simulink library "BLE_Library"  (R2017b)
settings: Solver=VariableStepAuto  StartTime=0.0  StopTime=10.0  RelTol=1e-3
values from neighbouring files (symbols this model uses):
  D = D/ScaleCoefficient    [BLE_PostLoad.m]    (also in new_BLE_model.m = zeros(N_BLE,N_BLE+1))
undefined symbols (not defined in the file or in its folder): ADV_IND_AccA, ADV_IND_id, BT_Hop_Separation, BT_Samples_Per_Symbol, CONNECT_IND_id, CONNECT_IND_length, F3B672D172DF, F506B10B1B3E, Header, LL_DATA_EMPTY_length, LL_DATA_id, magnitude, Payload, Preamble, Slot_Ts, T_IFS
libraries: BLE_Library x56, simulink x39, commutil2 x29, dspindex x17, commdigbbndfm2 x5, dspsigops x2, commrandsrc3 x2, dspstat3 x2, dspsrcs4 x1, dsparch4 x1, commdigbbndcpm2 x1
(part 2 of 5)

== system BLE_Library/CRC, Whitening, Modulation ==
  "Preamble, Access" : Inport
  "Header, Payload" : Inport  Port=2
  CRC_ini : Inport  Port=3
  ChIdx : Inport  Port=4
  Enable : EnablePort  StatesWhenEnabling=reset  ShowOutputPort=on
  CRC calculation : Subsystem  TreatAsAtomicUnit=on
  Compare To Constant : simulink/Logic and Bit Operations/Compare To Constant  relop=>  const=39  OutDataTypeStr=boolean
  Concatenate : Concatenate  Mode=Multidimensional array
  Counter Free-Running : simulink/Sources/Counter Free-Running  NumBits=32  tsamp=Slot_Ts
  Logical Operator1 : Logic  AllPortsSameDT=off  OutDataTypeStr=boolean
  Logical Operator2 : Logic  Operator=NOT  AllPortsSameDT=off  OutDataTypeStr=boolean
  Modulation : Subsystem
  Relational Operator1 : RelationalOperator  Operator=>  OutDataTypeStr=boolean  RndMeth=Simplest
  Selector1 : Subsystem
  Selector2 : Subsystem  TreatAsAtomicUnit=on
  Switch : Switch  Criteria=u2 > Threshold
  Switch1 : Switch  Criteria=u2 > Threshold
  Vector Concatenate1 : Concatenate
  Whitening : Subsystem
  Width1 : Width
  add CRC length : Bias  Bias=24
  TxBits : Outport  OutputWhenDisabled=reset  InitialOutput=0
  TxBitsLength : Outport  Port=2
  Tx signal : Outport  Port=3  OutputWhenDisabled=reset  InitialOutput=0
  wires:
  CRC_ini/1 -> CRC calculation/2(CRC_ini)
  "Preamble, Access"/1 -> Concatenate/1
  ChIdx/1 -> Whitening/2(ChIdx), Modulation/2(ChIdx)
  Counter Free-Running/1 -> Relational Operator1/2, Compare To Constant/1, Selector1/2(Idx)
  Concatenate/1 -> Width1/1, Selector1/1(U)
  "Header, Payload"/1 -> Concatenate/2
  Compare To Constant/1 -> Switch1/2, Whitening/Enable, Logical Operator1/2
  Width1/1 -> add CRC length/1, Relational Operator1/1
  Relational Operator1/1 -> Switch/2, Logical Operator2/1, Logical Operator1/1, Selector1/Enable
  Modulation/1(TxBits) -> Vector Concatenate1/1
  CRC calculation/1(CRC) -> Selector2/1(U)
  Switch1/1 -> Modulation/1(Tx bits)
  Enable/1 -> Vector Concatenate1/2
  Selector1/1(Out1) -> Switch1/3, Switch/1, CRC calculation/1(Payload)
  Logical Operator1/1 -> CRC calculation/Enable
  Selector2/1(Out1) -> Switch/3
  Logical Operator2/1 -> Selector2/Enable
  Modulation/2(Tx signal) -> Tx signal/1
  Vector Concatenate1/1 -> TxBits/1
  add CRC length/1 -> TxBitsLength/1
  Switch/1 -> Whitening/1(Payload)
  Whitening/1(Payload W) -> Switch1/1

== system BLE_Library/Channel ==

== system BLE_Library/Demodulation, De-whitening, CRC check, PDU ==
  Rx signal : Inport
  CRC_ini : Inport  Port=2
  AccA : Inport  Port=3
  ChIdx : Inport  Port=4
  Enable : EnablePort  StatesWhenEnabling=reset
  "Access Code check, Payload read enable" : Subsystem
  "De-whitening, CRC check, Data fields" : Subsystem
  Demodulation : Subsystem
  Terminator : Terminator
  AccA_OK : Outport
  CRC_OK : Outport  Port=2
  Payload_En : Outport  Port=3
  Header : Outport  Port=4
  PDU : Outport  Port=5
  RxBits : Outport  Port=6
  wires:
  "De-whitening, CRC check, Data fields"/3(PDU) -> PDU/1
  ChIdx/1 -> Demodulation/2(ChIdx), "De-whitening, CRC check, Data fields"/3(ChIdx)
  Demodulation/3(Rx bit 0) -> Terminator/1
  "De-whitening, CRC check, Data fields"/1(CRC_OK) -> CRC_OK/1
  Demodulation/1(Rx bit detected) -> "Access Code check, Payload read enable"/1(Rx bit detected)
  Demodulation/2(Rx bit 1) -> RxBits/1, "Access Code check, Payload read enable"/2(Rx bit 1), "De-whitening, CRC check, Data fields"/1(Paylaod W)
  Rx signal/1 -> Demodulation/1(Rx signal)
  "Access Code check, Payload read enable"/1(PayloadEn) -> "De-whitening, CRC check, Data fields"/Enable, Payload_En/1
  CRC_ini/1 -> "De-whitening, CRC check, Data fields"/2(CRC_ini)
  AccA/1 -> "Access Code check, Payload read enable"/3(AccA)
  "Access Code check, Payload read enable"/2(AccA_OK) -> AccA_OK/1
  "De-whitening, CRC check, Data fields"/2(Header) -> Header/1

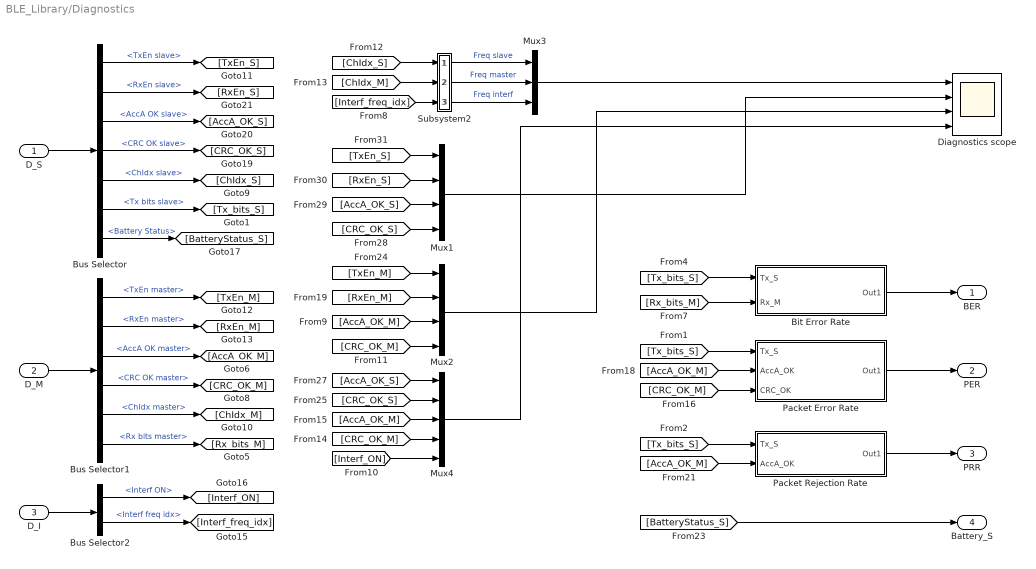
== system BLE_Library/Diagnostics ==
  D_S : Inport
  D_M : Inport  Port=2
  D_I : Inport  Port=3
  Bit Error Rate : Subsystem
      mask Display: disp('BER\n calculation')
  Bus Selector : BusSelector  OutputSignals=TxEn slave,RxEn slave,AccA OK slave,CRC OK slave,ChIdx slave,Tx bits slave,Battery Status
  Bus Selector1 : BusSelector  OutputSignals=TxEn master,RxEn master,AccA OK master,CRC OK master,ChIdx master,Rx bits master
  Bus Selector2 : BusSelector  OutputSignals=Interf ON,Interf freq idx
  Diagnostics scope : Scope  NumInputPorts=4
  Mux1 : Mux
  Mux2 : Mux
  Mux3 : Mux  Inputs=3
  Mux4 : Mux  Inputs=5
  Packet Error Rate : Subsystem
      mask Display: disp('PER\n calculation')
  Packet Rejection Rate : Subsystem
      mask Display: disp('PRR\n calculation')
  Subsystem2 : Subsystem
      mask Display: disp('')
  BER : Outport
  PER : Outport  Port=2
  PRR : Outport  Port=3
  Battery_S : Outport  Port=4
  wires:
  Mux4/1 -> Diagnostics scope/4
  Mux2/1 -> Diagnostics scope/3
  Mux1/1 -> Diagnostics scope/2
  Mux3/1 -> Diagnostics scope/1
  D_S/1 -> Bus Selector/1
  D_M/1 -> Bus Selector1/1
  Bit Error Rate/1(Out1) -> BER/1
  Bus Selector/6 -> [Tx_bits_S]  "<Tx bits slave>"
  [Tx_bits_S] -> Bit Error Rate/1(Tx_S)
  Bus Selector1/6 -> [Rx_bits_M]  "<Rx bits master>"
  [Rx_bits_M] -> Bit Error Rate/2(Rx_M)
  Bus Selector1/3 -> [AccA_OK_M]  "<AccA OK master>"
  Bus Selector1/4 -> [CRC_OK_M]  "<CRC OK master>"
  Bus Selector/5 -> [ChIdx_S]  "<ChIdx slave>"
  Bus Selector1/5 -> [ChIdx_M]  "<ChIdx master>"
  [CRC_OK_M] -> Mux4/4
  [AccA_OK_M] -> Packet Error Rate/2(AccA_OK)
  [CRC_OK_M] -> Packet Error Rate/3(CRC_OK)
  Packet Rejection Rate/1(Out1) -> PRR/1
  Bus Selector1/2 -> [RxEn_M]  "<RxEn master>"
  [RxEn_M] -> Mux2/2
  [AccA_OK_M] -> Packet Rejection Rate/2(AccA_OK)
  Packet Error Rate/1(Out1) -> PER/1
  [AccA_OK_M] -> Mux4/3
  [Interf_ON] -> Mux4/5
  [AccA_OK_M] -> Mux2/3
  [CRC_OK_M] -> Mux2/4
  [ChIdx_S] -> Subsystem2/1(In1)
  [ChIdx_M] -> Subsystem2/2(In2)
  [Interf_freq_idx] -> Subsystem2/3(In3)
  Subsystem2/1(Out1) -> Mux3/1  "Freq slave"
  Subsystem2/2(Out2) -> Mux3/2  "Freq master"
  Subsystem2/3(Out3) -> Mux3/3  "Freq interf"
  D_I/1 -> Bus Selector2/1
  Bus Selector2/1 -> [Interf_ON]  "<Interf ON>"
  Bus Selector2/2 -> [Interf_freq_idx]  "<Interf freq idx>"
  Bus Selector1/1 -> [TxEn_M]  "<TxEn master>"
  [TxEn_M] -> Mux2/1
  Bus Selector/4 -> [CRC_OK_S]  "<CRC OK slave>"
  [CRC_OK_S] -> Mux4/2
  Bus Selector/3 -> [AccA_OK_S]  "<AccA OK slave>"
  [AccA_OK_S] -> Mux4/1
  Bus Selector/2 -> [RxEn_S]  "<RxEn slave>"
  Bus Selector/1 -> [TxEn_S]  "<TxEn slave>"
  [AccA_OK_S] -> Mux1/3
  [CRC_OK_S] -> Mux1/4
  [RxEn_S] -> Mux1/2
  [TxEn_S] -> Mux1/1
  Bus Selector/7 -> [BatteryStatus_S]  "<Battery Status>"
  [BatteryStatus_S] -> Battery_S/1
  [Tx_bits_S] -> Packet Error Rate/1(Tx_S)
  [Tx_bits_S] -> Packet Rejection Rate/1(Tx_S)

== system BLE_Library/Export parameters ==

== system BLE_Library/Falling edge ==
  In1 : Inport
  Logical Operator3 : Logic  Operator=XOR  AllPortsSameDT=off  OutDataTypeStr=boolean
  Logical Operator4 : Logic  AllPortsSameDT=off  OutDataTypeStr=boolean
  Unit Delay1 : UnitDelay  SampleTime=Slot_Ts
  Out1 : Outport
  wires:
  In1/1 -> Logical Operator3/1, Unit Delay1/1
  Logical Operator4/1 -> Out1/1
  Unit Delay1/1 -> Logical Operator4/2, Logical Operator3/2
  Logical Operator3/1 -> Logical Operator4/1

== system BLE_Library/Packet Error Rate ==
  Tx_S : Inport
  AccA_OK : Inport  Port=2
  CRC_OK : Inport  Port=3
  Compare To Zero : simulink/Logic and Bit Operations/Compare To Zero  relop=>  OutDataTypeStr=boolean
  Constant : Constant  SampleTime=Slot_Ts
  Demux1 : Demux  Outputs=2
  Divide : Product  Inputs=*/
  Enabled Subsystem : Subsystem  TreatAsAtomicUnit=on
  Falling edge : BLE_Library/Falling edge  SystemSampleTime=-1
  Logical Operator : Logic  AllPortsSameDT=off  OutDataTypeStr=boolean
  Logical Operator2 : Logic  AllPortsSameDT=off  OutDataTypeStr=boolean
  Logical Operator3 : Logic  AllPortsSameDT=off  OutDataTypeStr=boolean
  Subsystem1 : BLE_Library/Subsystem2  offset=0
  Subsystem4 : BLE_Library/Subsystem2  offset=0
  Sum : Sum  Inputs=|-+
  Switch : Switch  Criteria=u2 > Threshold
  Terminator1 : Terminator
  Unit Delay1 : UnitDelay  SampleTime=Slot_Ts
  Unit Delay2 : UnitDelay  SampleTime=Slot_Ts
  Vector Concatenate1 : Concatenate  NumInputs=3
  Out1 : Outport
  wires:
  Constant/1 -> Switch/3
  Switch/1 -> Divide/2
  Compare To Zero/1 -> Logical Operator/2
  Logical Operator/1 -> Enabled Subsystem/Enable
  Falling edge/1 -> Logical Operator/1
  Sum/1 -> Divide/1, Vector Concatenate1/2
  Subsystem4/1 -> Sum/1
  Divide/1 -> Vector Concatenate1/1
  Subsystem1/1 -> Sum/2, Vector Concatenate1/3, Switch/1, Compare To Zero/1, Switch/2
  Vector Concatenate1/1 -> Enabled Subsystem/1(In1)
  Enabled Subsystem/1(Out1) -> Out1/1
  Tx_S/1 -> Unit Delay1/1
  Logical Operator2/1 -> Subsystem1/1
  Logical Operator3/1 -> Subsystem4/1
  Unit Delay2/1 -> Logical Operator2/2, Logical Operator3/1
  CRC_OK/1 -> Logical Operator3/2
  AccA_OK/1 -> Logical Operator2/1
  Unit Delay1/1 -> Demux1/1
  Demux1/1 -> Terminator1/1
  Demux1/2 -> Falling edge/1, Unit Delay2/1

== system BLE_Library/Packet Rejection Rate ==
  Tx_S : Inport
  AccA_OK : Inport  Port=2
  Compare To Zero1 : simulink/Logic and Bit Operations/Compare To Zero  relop=>  OutDataTypeStr=boolean
  Constant : Constant  SampleTime=Slot_Ts
  Demux : Demux  Outputs=2
  Divide1 : Product  Inputs=*/
  Enabled Subsystem1 : Subsystem  TreatAsAtomicUnit=on
  Falling edge : BLE_Library/Falling edge  SystemSampleTime=-1
  Logical Operator1 : Logic  AllPortsSameDT=off  OutDataTypeStr=boolean
  Logical Operator3 : Logic  AllPortsSameDT=off  OutDataTypeStr=boolean
  Rising edge : BLE_Library/Rising edge  SystemSampleTime=-1
  Subsystem1 : BLE_Library/Subsystem2  offset=0
  Subsystem4 : BLE_Library/Subsystem2  offset=0
  Sum1 : Sum  Inputs=|-+
  Switch : Switch  Criteria=u2 > Threshold
  Terminator : Terminator
  Unit Delay1 : UnitDelay  SampleTime=Slot_Ts
  Unit Delay2 : UnitDelay  SampleTime=Slot_Ts
  Vector Concatenate2 : Concatenate  NumInputs=3
  Out1 : Outport
  wires:
  Demux/2 -> Unit Delay1/1
  Demux/1 -> Terminator/1
  Tx_S/1 -> Demux/1
  Rising edge/1 -> Subsystem1/1
  Logical Operator3/1 -> Subsystem4/1
  AccA_OK/1 -> Logical Operator3/2
  Unit Delay2/1 -> Logical Operator3/1
  Unit Delay1/1 -> Rising edge/1, Unit Delay2/1, Falling edge/1
  Switch/1 -> Divide1/2
  Constant/1 -> Switch/3
  Compare To Zero1/1 -> Logical Operator1/2
  Vector Concatenate2/1 -> Enabled Subsystem1/1(In1)
  Divide1/1 -> Vector Concatenate2/1
  Subsystem1/1 -> Switch/2, Compare To Zero1/1, Switch/1, Vector Concatenate2/3, Sum1/2
  Falling edge/1 -> Logical Operator1/1
  Subsystem4/1 -> Sum1/1
  Sum1/1 -> Vector Concatenate2/2, Divide1/1
  Logical Operator1/1 -> Enabled Subsystem1/Enable
  Enabled Subsystem1/1(Out1) -> Out1/1

== system BLE_Library/Rising edge ==
  In1 : Inport
  Logical Operator3 : Logic  Operator=XOR  AllPortsSameDT=off  OutDataTypeStr=boolean
  Logical Operator4 : Logic  AllPortsSameDT=off  OutDataTypeStr=boolean
  Unit Delay1 : UnitDelay  SampleTime=Slot_Ts
  Out1 : Outport
  wires:
  In1/1 -> Logical Operator4/1, Logical Operator3/1, Unit Delay1/1
  Logical Operator4/1 -> Out1/1
  Unit Delay1/1 -> Logical Operator3/2
  Logical Operator3/1 -> Logical Operator4/2

== system BLE_Library/Sensor ==
  Integer to Bit Converter : commutil2/Integer to Bit Converter  nbits=NbitsPerSample  signedInputValues=Unsigned  bitOrder=MSB first  outDtype=boolean
  Rounding Function : Rounding  Operator=round
  Uniform Random Number : UniformRandomNumber  Minimum=0  Maximum=2^NbitsPerSample-1  SampleTime=Slot_Ts
  Out1 : Outport
  wires:
  Uniform Random Number/1 -> Rounding Function/1
  Rounding Function/1 -> Integer to Bit Converter/1
  Integer to Bit Converter/1 -> Out1/1

== system BLE_Library/Subsystem1 ==
  En_in : Inport
  PDU_type : Inport  Port=2
  Constant5 : Constant  Value=PDU_type  SampleTime=Slot_Ts
  Logical Operator3 : Logic  AllPortsSameDT=off  OutDataTypeStr=boolean
  Relational Operator3 : RelationalOperator  Operator===  OutDataTypeStr=boolean  RndMeth=Simplest
  En_out : Outport
  wires:
  PDU_type/1 -> Relational Operator3/2
  Logical Operator3/1 -> En_out/1
  Constant5/1 -> Relational Operator3/1
  En_in/1 -> Logical Operator3/1
  Relational Operator3/1 -> Logical Operator3/2

== system BLE_Library/Subsystem2 ==
  <CRC OK slave> : Inport
  Add1 : Sum  AccumDataTypeStr=uint32
  Add2 : Sum  Inputs=+-
  Constant : Constant  Value=offset  SampleTime=Slot_Ts
  Data Type Conversion1 : DataTypeConversion  OutDataTypeStr=double
  Unit Delay1 : UnitDelay  SampleTime=Slot_Ts
  Out1 : Outport
  wires:
  <CRC OK slave>/1 -> Data Type Conversion1/1
  Unit Delay1/1 -> Add1/1
  Add1/1 -> Add2/1, Unit Delay1/1
  Data Type Conversion1/1 -> Add1/2
  Add2/1 -> Out1/1
  Constant/1 -> Add2/2

== system BLE_Library/802.11b interferer/Enabled Subsystem ==
  In1 : Inport
  Enable : EnablePort  StatesWhenEnabling=reset
  Out3 : Outport  OutputWhenDisabled=reset  InitialOutput=0
  wires:
  In1/1 -> Out3/1

== system BLE_Library/802.11b interferer/Poisson pulses ==
  Constant5 : Constant  Value=1/average_rate-packet_length  SampleTime=Slot_Ts
  Constant6 : Constant  Value=0  SampleTime=Slot_Ts
  If : If  IfExpression=u1
  If Action Subsystem1 : Subsystem  TreatAsAtomicUnit=on
  If Action Subsystem2 : Subsystem  TreatAsAtomicUnit=on
  Merge : Merge
  Relational Operator1 : RelationalOperator  Operator=<=  OutDataTypeStr=boolean  RndMeth=Simplest
  enable : Outport
  wires:
  Constant6/1 -> Relational Operator1/2
  If/2 -> If Action Subsystem1/Action
  If/1 -> If Action Subsystem2/Action
  Relational Operator1/1 -> If/1
  Constant5/1 -> Relational Operator1/1
  If Action Subsystem2/1(enable) -> Merge/1
  If Action Subsystem1/1(enable) -> Merge/2
  Merge/1 -> enable/1

== system BLE_Library/BLE master/Master mode ==
  note: 1) Add Subsystem or Model blocks as valid variant choices.
      | 2) You cannot connect blocks at this level. At simulation, connectivity is automatically
      | determined, based on the active variant and port name matching.
  Turn ON : Inport
  Rx signal : Inport  Port=2
  In3 : Inport  Port=3
  Multiple slaves mode : Subsystem  VariantControl=MultipleSlavesMode
  One slave mode : Subsystem  VariantControl=OneSlaveMode
  Tx signal : Outport
  Diagnostics : Outport  Port=2

== system BLE_Library/BLE master/Subsystem7 ==
  In1 : Inport
  Compare To Zero : simulink/Logic and Bit Operations/Compare To Zero  relop=>  OutDataTypeStr=boolean
  Constant4 : Constant  Value=zeros(BT_Samples_Per_Symbol,1)  SampleTime=Slot_Ts
  Real-Imag to Complex : RealImagToComplex
  Step : Step  Time=3.492e-3  Before=1  After=0  SampleTime=Slot_Ts
  Step1 : Step  Time=3.55e-3  SampleTime=Slot_Ts
  Step2 : Step  Time=4060e-3  SampleTime=Slot_Ts
  Step5 : Step  Time=4020e-3  SampleTime=Slot_Ts
  Sum1 : Sum  Inputs=++-+
  Switch : Switch  Criteria=u2 > Threshold
  Out1 : Outport
  Out2 : Outport  Port=2
  wires:
  Compare To Zero/1 -> Out2/1
  Sum1/1 -> Switch/2, Compare To Zero/1
  Step/1 -> Sum1/1
  Step5/1 -> Sum1/3
  Step1/1 -> Sum1/2
  Switch/1 -> Out1/1
  In1/1 -> Switch/1
  Real-Imag to Complex/1 -> Switch/3
  Constant4/1 -> Real-Imag to Complex/2, Real-Imag to Complex/1
  Step2/1 -> Sum1/4

== system BLE_Library/BLE slave/ADV_IND ==
  Enable : EnablePort  StatesWhenEnabling=reset
  "ADV_IND Header, Payload" : Subsystem
  Subsystem4 : Subsystem
      mask Display: disp('Adv\nPreamble,\nAccess')
  "Preamble, Access" : Outport  InitialOutput=0
  "Header, Payload" : Outport  Port=2  InitialOutput=0
  wires:
  "ADV_IND Header, Payload"/1("Header, Payload") -> "Header, Payload"/1
  Subsystem4/1(Out1) -> "Preamble, Access"/1

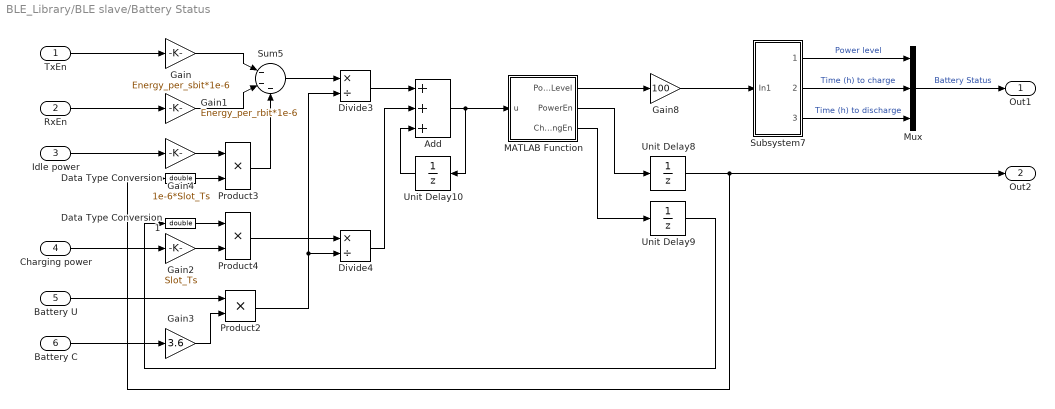
== system BLE_Library/BLE slave/Battery Status ==
  TxEn : Inport
  RxEn : Inport  Port=2
  Idle power : Inport  Port=3
  Charging power : Inport  Port=4
  Battery U : Inport  Port=5
  Battery C : Inport  Port=6
  Add : Sum  Inputs=+++
  Data Type Conversion : DataTypeConversion  OutDataTypeStr=double
  Data Type Conversion1 : DataTypeConversion  OutDataTypeStr=double
  Divide3 : Product  Inputs=*/
  Divide4 : Product  Inputs=*/
  Gain : Gain  Gain=Energy_per_sbit*1e-6
  Gain1 : Gain  Gain=Energy_per_rbit*1e-6
  Gain2 : Gain  Gain=Slot_Ts
  Gain3 : Gain  Gain=3.6
  Gain4 : Gain  Gain=1e-6*Slot_Ts
  Gain8 : Gain  Gain=100
  MATLAB Function : MATLAB Function  TreatAsAtomicUnit=on
  Mux : Mux  Inputs=3
  Product2 : Product
  Product3 : Product
  Product4 : Product
  Subsystem7 : Subsystem
      mask Display: disp('Battery\nStatus')
  Sum5 : Sum  Inputs=|---
  Unit Delay10 : UnitDelay  InitialCondition=1  SampleTime=Slot_Ts
  Unit Delay8 : UnitDelay  SampleTime=Slot_Ts
  Unit Delay9 : UnitDelay  SampleTime=Slot_Ts
  Out1 : Outport
  Out2 : Outport  Port=2
  wires:
  Mux/1 -> Out1/1  "Battery Status"
  TxEn/1 -> Gain/1
  RxEn/1 -> Gain1/1
  Idle power/1 -> Gain4/1
  Product3/1 -> Sum5/3
  Product2/1 -> Divide4/2, Divide3/2
  Battery U/1 -> Product2/1
  Gain4/1 -> Product3/1
  Battery C/1 -> Gain3/1
  Gain3/1 -> Product2/2
  Unit Delay8/1 -> Out2/1, Data Type Conversion/1
  Data Type Conversion/1 -> Product3/2
  Gain8/1 -> Subsystem7/1(In1)
  MATLAB Function/2(PowerEn) -> Unit Delay8/1
  MATLAB Function/3(ChargingEn) -> Unit Delay9/1
  Charging power/1 -> Gain2/1
  Gain/1 -> Sum5/1
  Gain1/1 -> Sum5/2
  Unit Delay9/1 -> Data Type Conversion1/1
  Sum5/1 -> Divide3/1
  Product4/1 -> Divide4/1
  MATLAB Function/1(PowerLevel) -> Gain8/1
  Data Type Conversion1/1 -> Product4/1
  Gain2/1 -> Product4/2
  Divide3/1 -> Add/1
  Divide4/1 -> Add/2
  Add/1 -> Unit Delay10/1, MATLAB Function/1(u)
  Unit Delay10/1 -> Add/3
  Subsystem7/3(Time (h) to discharge) -> Mux/3  "Time (h) to discharge"
  Subsystem7/2(Time (h) to charge) -> Mux/2  "Time (h) to charge"
  Subsystem7/1(Power level) -> Mux/1  "Power level"

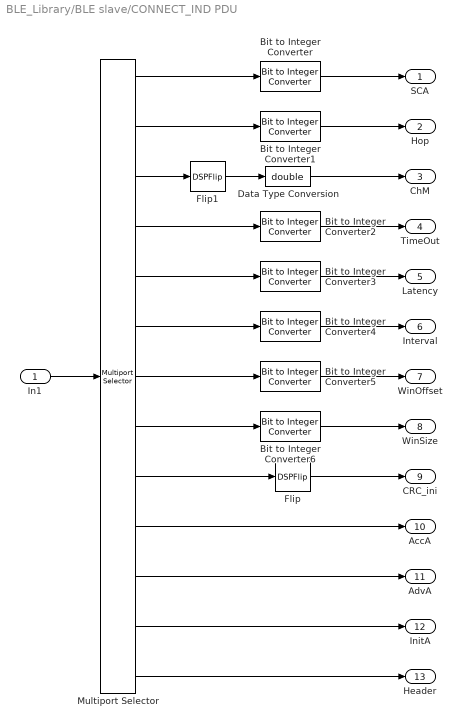
== system BLE_Library/BLE slave/CONNECT_IND PDU ==
  In1 : Inport  OutDataTypeStr=boolean
  Bit to Integer Converter : commutil2/Bit to Integer Converter  nbits=3  bitOrder=MSB first  signedOutputValues=Unsigned  outDtype=double  outDtypeSigned=Inherit via internal rule
  Bit to Integer Converter1 : commutil2/Bit to Integer Converter  nbits=5  bitOrder=MSB first  signedOutputValues=Unsigned  outDtype=double  outDtypeSigned=Inherit via internal rule
  Bit to Integer Converter{2..5} (4 alike) : commutil2/Bit to Integer Converter  nbits=16  bitOrder=MSB first  signedOutputValues=Unsigned  outDtype=double  outDtypeSigned=Inherit via internal rule
  Bit to Integer Converter6 : commutil2/Bit to Integer Converter  nbits=8  bitOrder=MSB first  signedOutputValues=Unsigned  outDtype=double  outDtypeSigned=Inherit via internal rule
  Data Type Conversion : DataTypeConversion  OutDataTypeStr=double
  Flip : DSPFlip
  Flip1 : DSPFlip
  Multiport Selector : dspindex/Multiport Selector  rowsOrCols=Rows  idxCellArray={1:3,4:8,9:48,49:64,65:80,81:96,97:112,113:120,121:144,145:176,177:224,225:272,273:288}  idxErrMode=Clip Index
  SCA : Outport
  Hop : Outport  Port=2
  ChM : Outport  Port=3
  TimeOut : Outport  Port=4
  Latency : Outport  Port=5
  Interval : Outport  Port=6
  WinOffset : Outport  Port=7
  WinSize : Outport  Port=8
  CRC_ini : Outport  Port=9
  AccA : Outport  Port=10
  AdvA : Outport  Port=11
  InitA : Outport  Port=12
  Header : Outport  Port=13
  wires:
  Flip1/1 -> Data Type Conversion/1
  Flip/1 -> CRC_ini/1
  Data Type Conversion/1 -> ChM/1
  Bit to Integer Converter6/1 -> WinSize/1
  Bit to Integer Converter5/1 -> WinOffset/1
  Bit to Integer Converter4/1 -> Interval/1
  Bit to Integer Converter3/1 -> Latency/1
  Bit to Integer Converter2/1 -> TimeOut/1
  Bit to Integer Converter1/1 -> Hop/1
  Bit to Integer Converter/1 -> SCA/1
  Multiport Selector/13 -> Header/1
  Multiport Selector/12 -> InitA/1
  Multiport Selector/11 -> AdvA/1
  Multiport Selector/10 -> AccA/1
  Multiport Selector/9 -> Flip/1
  Multiport Selector/8 -> Bit to Integer Converter6/1
  Multiport Selector/7 -> Bit to Integer Converter5/1
  Multiport Selector/6 -> Bit to Integer Converter4/1
  Multiport Selector/5 -> Bit to Integer Converter3/1
  Multiport Selector/4 -> Bit to Integer Converter2/1
  Multiport Selector/3 -> Flip1/1
  Multiport Selector/2 -> Bit to Integer Converter1/1
  Multiport Selector/1 -> Bit to Integer Converter/1
  In1/1 -> Multiport Selector/1

== system BLE_Library/BLE slave/LL_DATA ==
  Access : Inport
  MD_SN_NESN : Inport  Port=2
  Data : Inport  Port=3
  Enable : EnablePort  StatesWhenEnabling=reset
  "Concatenate Preamble, Access address" : Concatenate  Mode=Multidimensional array
  Fcn : Fcn  Expr=u/8
  Flip : DSPFlip
  Flip1 : DSPFlip
  Header : Concatenate  NumInputs=4  Mode=Multidimensional array
  Header and Payload : Concatenate  Mode=Multidimensional array
  Integer to Bit Converter3 : commutil2/Integer to Bit Converter  nbits=8  signedInputValues=Unsigned  bitOrder=MSB first  outDtype=boolean
  LLID : Constant  Value=[0 1]'  OutDataTypeStr=boolean  SampleTime=Slot_Ts
  MATLAB Function : MATLAB Function  TreatAsAtomicUnit=on
  RFU : Constant  Value=[0 0 0]'  OutDataTypeStr=boolean  SampleTime=Slot_Ts
  Width : Width
  "Preamble, Access" : Outport  InitialOutput=0
  "Header, Payload" : Outport  Port=2  InitialOutput=0
  wires:
  Data/1 -> Header and Payload/2, Width/1
  Flip1/1 -> Header/4
  RFU/1 -> Header/3
  Flip/1 -> Header/2
  MD_SN_NESN/1 -> Flip/1
  Header/1 -> Header and Payload/1
  Header and Payload/1 -> "Header, Payload"/1
  Integer to Bit Converter3/1 -> Flip1/1
  Width/1 -> Fcn/1
  Fcn/1 -> Integer to Bit Converter3/1
  LLID/1 -> Header/1
  "Concatenate Preamble, Access address"/1 -> "Preamble, Access"/1
  MATLAB Function/1(Preamble) -> "Concatenate Preamble, Access address"/1
  Access/1 -> MATLAB Function/1(AccessAddress), "Concatenate Preamble, Access address"/2

== system BLE_Library/BLE slave/Subsystem ==
  Data in : Inport
  Enable : EnablePort  StatesWhenEnabling=reset
  Data out : Outport
  wires:
  Data in/1 -> Data out/1

== system BLE_Library/BLE slave/Subsystem3 ==
  In1 : Inport
  Constant4 : Constant  Value=zeros(BT_Samples_Per_Symbol,1)  SampleTime=Slot_Ts
  Real-Imag to Complex : RealImagToComplex
  Step2 : Step  Time=10e-3  Before=1  After=0  SampleTime=Slot_Ts
  Step3 : Step  Time=3500  SampleTime=Slot_Ts
  Sum2 : Sum  Inputs=|++
  Switch : Switch  Criteria=u2 > Threshold
  Out1 : Outport
  wires:
  Constant4/1 -> Real-Imag to Complex/1, Real-Imag to Complex/2
  Real-Imag to Complex/1 -> Switch/3
  Step3/1 -> Sum2/1
  Step2/1 -> Sum2/2
  Sum2/1 -> Switch/2
  In1/1 -> Switch/1
  Switch/1 -> Out1/1

== system BLE_Library/BLE slave/Subsystem5 ==
  AdvA : Inport
  InitA : Inport  Port=2
  Compare To Constant1 : simulink/Logic and Bit Operations/Compare To Constant  relop===  const=1  OutDataTypeStr=boolean
  Constant1 : Constant  Value=PDU_Type  VectorParams1D=off  OutDataTypeStr=double  SampleTime=Slot_Ts
  If : If  IfExpression=u1
  If Action Subsystem : Subsystem  TreatAsAtomicUnit=on
  If Action Subsystem1 : Subsystem  TreatAsAtomicUnit=on
  Merge2 : Merge
  CON OK : Outport
  wires:
  If/2 -> If Action Subsystem1/Action
  AdvA/1 -> If Action Subsystem1/1(AdvA), If Action Subsystem/1(AdvA)
  InitA/1 -> If Action Subsystem1/2(InitA)
  If/1 -> If Action Subsystem/Action
  If Action Subsystem1/1(CON OK) -> Merge2/2
  If Action Subsystem/1(CON OK) -> Merge2/1
  Merge2/1 -> CON OK/1
  Constant1/1 -> Compare To Constant1/1
  Compare To Constant1/1 -> If/1

== system BLE_Library/BLE slave/Subsystem7 ==
  In1 : Inport
  Compare To Zero : simulink/Logic and Bit Operations/Compare To Zero  relop=>  OutDataTypeStr=boolean
  Constant4 : Constant  Value=zeros(BT_Samples_Per_Symbol,1)  SampleTime=Slot_Ts
  Real-Imag to Complex : RealImagToComplex
  Step : Step  Time=3.74e-3  Before=1  After=0  SampleTime=Slot_Ts
  Step1 : Step  Time=3.75e-3  SampleTime=Slot_Ts
  Step2 : Step  Time=4.78e-3  SampleTime=Slot_Ts
  Step5 : Step  Time=4.16e-3  SampleTime=Slot_Ts
  Sum1 : Sum  Inputs=++-+
  Switch : Switch  Criteria=u2 > Threshold
  Out1 : Outport
  Out2 : Outport  Port=2
  wires:
  Constant4/1 -> Real-Imag to Complex/1, Real-Imag to Complex/2
  Real-Imag to Complex/1 -> Switch/3
  In1/1 -> Switch/1
  Switch/1 -> Out1/1
  Step1/1 -> Sum1/2
  Step5/1 -> Sum1/3
  Step/1 -> Sum1/1
  Sum1/1 -> Compare To Zero/1, Switch/2
  Compare To Zero/1 -> Out2/1
  Step2/1 -> Sum1/4

== system BLE_Library/Bit Error Rate/Enabled Subsystem1 ==
  In1 : Inport
  Enable : EnablePort
  Out1 : Outport
  wires:
  In1/1 -> Out1/1

== system BLE_Library/CRC, Whitening, Modulation/CRC calculation ==
  Payload : Inport
  CRC_ini : Inport  Port=2
  Enable : EnablePort  StatesWhenEnabling=reset
  CRC generation : MATLAB Function  TreatAsAtomicUnit=on
  Constant3 : Constant  SampleTime=Slot_Ts
  Flip : DSPFlip
  Switch : Switch  Criteria=u2 > Threshold
  Unit Delay1 : UnitDelay  SampleTime=Slot_Ts
  Unit Delay8 : UnitDelay  SampleTime=Slot_Ts
  CRC : Outport
  wires:
  Payload/1 -> CRC generation/1(bin)
  Unit Delay1/1 -> Switch/2
  Constant3/1 -> Unit Delay1/1
  CRC generation/1(CRC) -> Unit Delay8/1, Flip/1
  CRC_ini/1 -> Switch/3
  Unit Delay8/1 -> Switch/1
  Switch/1 -> CRC generation/2(LFSR)
  Flip/1 -> CRC/1

== system BLE_Library/CRC, Whitening, Modulation/Modulation ==
  Tx bits : Inport
  ChIdx : Inport  Port=2
  GFSK Modulation : commdigbbndcpm2/CPM Modulator Baseband  Mnum=2  inputType=Bit  mappingType=Binary  modIdx=0.5  pulseShape=Gaussian  BT=0.5  mainLobePulseLength=1  rollOff=0.2  pulseLength=1  preHistory=1  phaseOffset=0  samplesPerSymbol=BT_Samples_Per_Symbol  RateOptions=Enforce single-rate processing  outDataType=double
      settings: SourceProductName=Communications System Toolbox  SourceProductBaseCode=CM
  Look-Up Table : Lookup  InputValues=0:39  Table=[1:11 13:38 0 12 39]  SaturateOnIntegerOverflow=on
  M-FSK Modulator Baseband : commdigbbndfm2/M-FSK Modulator Baseband  M=Num_Hop_Frequencies  InType=Integer  Enc=Binary  freqSep=BT_Hop_Separation  phaseType=Continuous  numSamp=BT_Samples_Per_Symbol  RateOptions=Enforce single-rate processing  outDataType=double
      settings: SourceProductName=Communications System Toolbox
  Mix to appropriate hop frequency : Product  SaturateOnIntegerOverflow=on  InputSameDT=on  OutDataTypeStr=Inherit: Same as first input
  TxBits : Outport  OutputWhenDisabled=reset  InitialOutput=0
  Tx signal : Outport  Port=2  OutputWhenDisabled=reset  InitialOutput=0
  wires:
  GFSK Modulation/1 -> Mix to appropriate hop frequency/1
  ChIdx/1 -> Look-Up Table/1
  Tx bits/1 -> GFSK Modulation/1, TxBits/1
  Mix to appropriate hop frequency/1 -> Tx signal/1
  M-FSK Modulator Baseband/1 -> Mix to appropriate hop frequency/2
  Look-Up Table/1 -> M-FSK Modulator Baseband/1

== system BLE_Library/CRC, Whitening, Modulation/Selector1 ==
  U : Inport
  Idx : Inport  Port=2
  Enable : EnablePort  StatesWhenEnabling=reset
  Selector : Selector  NumberOfDimensions=2  IndexMode=Zero-based  InputPortWidth=3  IndexOptions=Index vector (port),Index vector (dialog)  Indices=0,0  OutputSizes=1,1
  Out1 : Outport
  wires:
  U/1 -> Selector/1
  Idx/1 -> Selector/2
  Selector/1 -> Out1/1

== system BLE_Library/CRC, Whitening, Modulation/Selector2 ==
  U : Inport
  Enable : EnablePort  StatesWhenEnabling=reset
  Counter Free-Running : simulink/Sources/Counter Free-Running  NumBits=32  tsamp=Slot_Ts
  Selector : Selector  NumberOfDimensions=2  IndexMode=Zero-based  InputPortWidth=3  IndexOptions=Index vector (dialog),Index vector (port)  Indices=0,0  OutputSizes=1,1
  Out1 : Outport
  wires:
  U/1 -> Selector/1
  Selector/1 -> Out1/1
  Counter Free-Running/1 -> Selector/2

== system BLE_Library/CRC, Whitening, Modulation/Whitening ==
  Payload : Inport
  ChIdx : Inport  Port=2
  Enable : EnablePort  StatesWhenEnabling=reset
  Constant3 : Constant  SampleTime=Slot_Ts
  Initial LFSR : Subsystem
  Switch : Switch  Criteria=u2 > Threshold
  Unit Delay1 : UnitDelay  SampleTime=Slot_Ts
  Unit Delay8 : UnitDelay  SampleTime=Slot_Ts
  Whitening : MATLAB Function  TreatAsAtomicUnit=on
  Payload W : Outport
  wires:
  Unit Delay1/1 -> Switch/2
  Whitening/1(bout) -> Payload W/1
  Payload/1 -> Whitening/1(bin)
  Initial LFSR/1(LFSR) -> Switch/3
  Constant3/1 -> Initial LFSR/Enable, Unit Delay1/1
  Switch/1 -> Whitening/2(LFSR)
  ChIdx/1 -> Initial LFSR/1(ChIdx)
  Unit Delay8/1 -> Switch/1
  Whitening/2(LFSR_new) -> Unit Delay8/1

== system BLE_Library/Demodulation, De-whitening, CRC check, PDU/Access Code check, Payload read enable ==
  note: Rising edge pulse
  Rx bit detected : Inport
  Rx bit 1 : Inport  Port=2
  AccA : Inport  Port=3
  AccA check : Subsystem
  Logical Operator3 : Logic  Operator=XOR  AllPortsSameDT=off  OutDataTypeStr=boolean
  Logical Operator4 : Logic  AllPortsSameDT=off  OutDataTypeStr=boolean
  Payload read enable : Stateflow chart  TreatAsAtomicUnit=on
  Unit Delay1 : UnitDelay  SampleTime=Slot_Ts
  Unit Delay2 : UnitDelay  SampleTime=Slot_Ts
  PayloadEn : Outport
  AccA_OK : Outport  Port=2
  wires:
  AccA check/1(AccA OK) -> Unit Delay2/1, Logical Operator3/1, Logical Operator4/1
  Unit Delay2/1 -> Logical Operator3/2
  Logical Operator3/1 -> Logical Operator4/2
  Rx bit detected/1 -> AccA check/Enable, Payload read enable/1(DataEn)
  Rx bit 1/1 -> AccA check/1(Rx bits)
  AccA/1 -> AccA check/2(AccA)
  Logical Operator4/1 -> AccA_OK/1, Payload read enable/2(AccA_OK)
  Payload read enable/1(PayloadEn) -> Unit Delay1/1
  Unit Delay1/1 -> PayloadEn/1

== system BLE_Library/Demodulation, De-whitening, CRC check, PDU/De-whitening, CRC check, Data fields ==
  Paylaod W : Inport
  CRC_ini : Inport  Port=2
  ChIdx : Inport  Port=3
  Enable : EnablePort  StatesWhenEnabling=reset
  Bias : Bias  Bias=15
  CRC calculation1 : Subsystem  TreatAsAtomicUnit=on
  CRC comparison : Subsystem  TreatAsAtomicUnit=on
  Compare To Constant : simulink/Logic and Bit Operations/Compare To Constant  relop===  const=15  OutDataTypeStr=boolean
  Compare To Constant1 : simulink/Logic and Bit Operations/Compare To Constant  relop=<  const=16  OutDataTypeStr=boolean
  Counter Free-Running : simulink/Sources/Counter Free-Running  NumBits=32  tsamp=Slot_Ts
  Data : Subsystem  TreatAsAtomicUnit=on
  De-whitening : Subsystem
  Get length : Subsystem  TreatAsAtomicUnit=on
  Logical Operator : Logic  Operator=NOT  AllPortsSameDT=off  OutDataTypeStr=boolean
  Relational Operator : RelationalOperator  Operator===  OutDataTypeStr=boolean  RndMeth=Simplest
  Relational Operator3 : RelationalOperator  Operator=<=  OutDataTypeStr=boolean  RndMeth=Simplest
  Store header : Subsystem  TreatAsAtomicUnit=on
  Tapped Delay3 : simulink/Discrete/Tapped Delay  vinit=0  samptime=Slot_Ts  NumDelays=PDU_Length-1  DelayOrder=Newest  includeCurrent=on
  CRC_OK : Outport  OutputWhenDisabled=reset  InitialOutput=0
  Header : Outport  Port=2
  PDU : Outport  Port=3  InitialOutput=0
  wires:
  Bias/1 -> Relational Operator/1, Relational Operator3/2
  Compare To Constant/1 -> Get length/Enable
  Get length/1(L) -> Bias/1
  ChIdx/1 -> De-whitening/2(ChIdx)
  Paylaod W/1 -> De-whitening/1(Payload W)
  Logical Operator/1 -> CRC comparison/Enable
  Relational Operator3/1 -> CRC calculation1/Enable, Logical Operator/1
  CRC comparison/1(CRC_OK) -> CRC_OK/1
  Store header/1(H) -> Get length/1(In1)
  CRC calculation1/1(CRC) -> CRC comparison/1(CRC calculated)
  CRC_ini/1 -> CRC calculation1/2(CRC_ini)
  Get length/2(H) -> Header/1
  Compare To Constant1/1 -> Store header/Enable
  Counter Free-Running/1 -> Relational Operator/2, Compare To Constant1/1, Compare To Constant/1, Relational Operator3/1
  Data/1(PDU) -> PDU/1
  Tapped Delay3/1 -> Data/1(In1)
  Relational Operator/1 -> Data/Enable
  De-whitening/1(Payload) -> Store header/1(P), CRC calculation1/1(Payload), Tapped Delay3/1, CRC comparison/2(CRC received)

== system BLE_Library/Demodulation, De-whitening, CRC check, PDU/Demodulation ==
  Rx signal : Inport
  ChIdx : Inport  Port=2
  Constant1 : Constant  Value=0  SampleTime=Slot_Ts
  Constant2 : Constant  SampleTime=Slot_Ts
  Logical Operator : Logic  Operator=OR  AllPortsSameDT=off  OutDataTypeStr=boolean
  Look-Up Table : Lookup  InputValues=0:39  Table=[1:11 13:38 0 12 39]  SaturateOnIntegerOverflow=on
  M-FSK Modulator Baseband1 : commdigbbndfm2/M-FSK Modulator Baseband  M=Num_Hop_Frequencies  InType=Integer  Enc=Binary  freqSep=BT_Hop_Separation  phaseType=Continuous  numSamp=BT_Samples_Per_Symbol  RateOptions=Enforce single-rate processing  outDataType=double
      settings: SourceProductName=Communications System Toolbox
  M-FSK Modulator Baseband2 : commdigbbndfm2/M-FSK Modulator Baseband  M=2  InType=Integer  Enc=Binary  freqSep=BT_Freq_Deviation  phaseType=Continuous  numSamp=BT_Samples_Per_Symbol  RateOptions=Enforce single-rate processing  outDataType=double  mask(M-FSK Modulator Baseband){}
      settings: SourceProductName=Communications System Toolbox
  M-FSK Modulator Baseband3 : commdigbbndfm2/M-FSK Modulator Baseband  M=2  InType=Integer  Enc=Binary  freqSep=BT_Freq_Deviation  phaseType=Continuous  numSamp=BT_Samples_Per_Symbol  RateOptions=Enforce single-rate processing  outDataType=double  mask(M-FSK Modulator Baseband){}
      settings: SourceProductName=Communications System Toolbox
  Math Function1 : Math  Operator=magnitude^2  SaturateOnIntegerOverflow=on
  Math Function2 : Math  Operator=conj  SaturateOnIntegerOverflow=on
  Math Function3 : Math  Operator=conj  SaturateOnIntegerOverflow=on
  Math Function4 : Math  Operator=magnitude^2  SaturateOnIntegerOverflow=on
  Math Function5 : Math  Operator=conj  SaturateOnIntegerOverflow=on
  Mean : dspstat3/Mean  run=off  reset_popup=None  InputProcessing=Columns as channels (frame based)  directionMode=Entire input  dimension=1  roiEnable=off  roiType=Rectangles  roiPortion=Entire ROI  roiOutput=Individual statistics for each ROI  roiFlag=off  outputDataTypeStr=Inherit: Same as accumulator  outputLastDataTypeStr=Inherit: Same as accumulator  outputMin=[]  outputMax=[]  roundingMode=Floor  overflowMode=off
  Mean1 : dspstat3/Mean  run=off  reset_popup=None  InputProcessing=Columns as channels (frame based)  directionMode=Entire input  dimension=1  roiEnable=off  roiType=Rectangles  roiPortion=Entire ROI  roiOutput=Individual statistics for each ROI  roiFlag=off  outputDataTypeStr=Inherit: Same as accumulator  outputLastDataTypeStr=Inherit: Same as accumulator  outputMin=[]  outputMax=[]  roundingMode=Floor  overflowMode=off
  Product1 : Product  SaturateOnIntegerOverflow=on  InputSameDT=on  OutDataTypeStr=Inherit: Same as first input
  Product3 : Product
  Product4 : Product
  Relational Operator : RelationalOperator  Operator=>  OutDataTypeStr=boolean  RndMeth=Simplest
  Relational Operator1 : RelationalOperator  OutDataTypeStr=boolean  RndMeth=Simplest
  Rx bit detected : Outport
  Rx bit 1 : Outport  Port=2
  Rx bit 0 : Outport  Port=3
  wires:
  Product3/1 -> Mean/1
  Logical Operator/1 -> Rx bit detected/1
  Math Function5/1 -> Product1/2
  M-FSK Modulator Baseband1/1 -> Math Function5/1
  Relational Operator/1 -> Rx bit 0/1, Logical Operator/1
  Relational Operator1/1 -> Rx bit 1/1, Logical Operator/2
  Constant1/1 -> M-FSK Modulator Baseband2/1
  Math Function1/1 -> Relational Operator/1, Relational Operator1/2
  Math Function4/1 -> Relational Operator1/1, Relational Operator/2
  Math Function2/1 -> Product3/2
  Product4/1 -> Mean1/1
  M-FSK Modulator Baseband2/1 -> Math Function2/1
  Math Function3/1 -> Product4/2
  M-FSK Modulator Baseband3/1 -> Math Function3/1
  Constant2/1 -> M-FSK Modulator Baseband3/1
  Mean1/1 -> Math Function4/1
  Mean/1 -> Math Function1/1
  Rx signal/1 -> Product1/1
  Product1/1 -> Product4/1, Product3/1
  ChIdx/1 -> Look-Up Table/1
  Look-Up Table/1 -> M-FSK Modulator Baseband1/1

== system BLE_Library/Diagnostics/Bit Error Rate ==
  Tx_S : Inport
  Rx_M : Inport  Port=2
  Compare To Zero1 : simulink/Logic and Bit Operations/Compare To Zero  relop=>  OutDataTypeStr=boolean
  Constant : Constant  SampleTime=Slot_Ts
  Demux : Demux  Outputs=2
  Demux1 : Demux  Outputs=2
  Divide1 : Product  Inputs=*/
  Enabled Subsystem1 : Subsystem  TreatAsAtomicUnit=on
  Falling edge : BLE_Library/Falling edge  SystemSampleTime=-1
  Logical Operator : Logic  Operator=NXOR  AllPortsSameDT=off  OutDataTypeStr=boolean
  Logical Operator1 : Logic  AllPortsSameDT=off  OutDataTypeStr=boolean
  Logical Operator3 : Logic  AllPortsSameDT=off  OutDataTypeStr=boolean
  Subsystem4 : BLE_Library/Subsystem2  offset=0
  Subsystem7 : BLE_Library/Subsystem2  offset=0
  Sum1 : Sum  Inputs=|-+
  Switch : Switch  Criteria=u2 > Threshold
  Terminator : Terminator
  Unit Delay1 : UnitDelay  SampleTime=Slot_Ts
  Vector Concatenate2 : Concatenate  NumInputs=3
  Out1 : Outport
  wires:
  Demux1/1 -> Logical Operator/1
  Demux/1 -> Logical Operator/2
  Unit Delay1/1 -> Demux/1
  Demux1/2 -> Terminator/1
  Logical Operator1/1 -> Subsystem7/1
  Tx_S/1 -> Unit Delay1/1
  Demux/2 -> Subsystem4/1, Falling edge/1, Logical Operator1/2
  Logical Operator/1 -> Logical Operator1/1
  Rx_M/1 -> Demux1/1
  Switch/1 -> Divide1/2
  Constant/1 -> Switch/3
  Compare To Zero1/1 -> Logical Operator3/2
  Vector Concatenate2/1 -> Enabled Subsystem1/1(In1)
  Divide1/1 -> Vector Concatenate2/1
  Subsystem4/1 -> Switch/2, Compare To Zero1/1, Switch/1, Vector Concatenate2/3, Sum1/2
  Falling edge/1 -> Logical Operator3/1
  Subsystem7/1 -> Sum1/1
  Sum1/1 -> Vector Concatenate2/2, Divide1/1
  Logical Operator3/1 -> Enabled Subsystem1/Enable
  Enabled Subsystem1/1(Out1) -> Out1/1

== system BLE_Library/Diagnostics/Packet Error Rate ==
  Tx_S : Inport
  AccA_OK : Inport  Port=2
  CRC_OK : Inport  Port=3
  Compare To Zero : simulink/Logic and Bit Operations/Compare To Zero  relop=>  OutDataTypeStr=boolean
  Constant : Constant  SampleTime=Slot_Ts
  Demux1 : Demux  Outputs=2
  Divide : Product  Inputs=*/
  Enabled Subsystem : Subsystem  TreatAsAtomicUnit=on
  Falling edge : BLE_Library/Falling edge  SystemSampleTime=-1
  Logical Operator : Logic  AllPortsSameDT=off  OutDataTypeStr=boolean
  Logical Operator2 : Logic  AllPortsSameDT=off  OutDataTypeStr=boolean
  Logical Operator3 : Logic  AllPortsSameDT=off  OutDataTypeStr=boolean
  Subsystem1 : BLE_Library/Subsystem2  offset=0
  Subsystem4 : BLE_Library/Subsystem2  offset=0
  Sum : Sum  Inputs=|-+
  Switch : Switch  Criteria=u2 > Threshold
  Terminator1 : Terminator
  Unit Delay1 : UnitDelay  SampleTime=Slot_Ts
  Unit Delay2 : UnitDelay  SampleTime=Slot_Ts
  Vector Concatenate1 : Concatenate  NumInputs=3
  Out1 : Outport
  wires:
  Constant/1 -> Switch/3
  Switch/1 -> Divide/2
  Compare To Zero/1 -> Logical Operator/2
  Logical Operator/1 -> Enabled Subsystem/Enable
  Falling edge/1 -> Logical Operator/1
  Sum/1 -> Divide/1, Vector Concatenate1/2
  Subsystem4/1 -> Sum/1
  Divide/1 -> Vector Concatenate1/1
  Subsystem1/1 -> Sum/2, Vector Concatenate1/3, Switch/1, Compare To Zero/1, Switch/2
  Vector Concatenate1/1 -> Enabled Subsystem/1(In1)
  Enabled Subsystem/1(Out1) -> Out1/1
  Tx_S/1 -> Unit Delay1/1
  Logical Operator2/1 -> Subsystem1/1
  Logical Operator3/1 -> Subsystem4/1
  Unit Delay2/1 -> Logical Operator2/2, Logical Operator3/1
  CRC_OK/1 -> Logical Operator3/2
  AccA_OK/1 -> Logical Operator2/1
  Unit Delay1/1 -> Demux1/1
  Demux1/1 -> Terminator1/1
  Demux1/2 -> Falling edge/1, Unit Delay2/1

== system BLE_Library/Diagnostics/Packet Rejection Rate ==
  Tx_S : Inport
  AccA_OK : Inport  Port=2
  Compare To Zero1 : simulink/Logic and Bit Operations/Compare To Zero  relop=>  OutDataTypeStr=boolean
  Constant : Constant  SampleTime=Slot_Ts
  Demux : Demux  Outputs=2
  Divide1 : Product  Inputs=*/
  Enabled Subsystem1 : Subsystem  TreatAsAtomicUnit=on
  Falling edge : BLE_Library/Falling edge  SystemSampleTime=-1
  Logical Operator1 : Logic  AllPortsSameDT=off  OutDataTypeStr=boolean
  Logical Operator3 : Logic  AllPortsSameDT=off  OutDataTypeStr=boolean
  Rising edge : BLE_Library/Rising edge  SystemSampleTime=-1
  Subsystem1 : BLE_Library/Subsystem2  offset=0
  Subsystem4 : BLE_Library/Subsystem2  offset=0
  Sum1 : Sum  Inputs=|-+
  Switch : Switch  Criteria=u2 > Threshold
  Terminator : Terminator
  Unit Delay1 : UnitDelay  SampleTime=Slot_Ts
  Unit Delay2 : UnitDelay  SampleTime=Slot_Ts
  Vector Concatenate2 : Concatenate  NumInputs=3
  Out1 : Outport
  wires:
  Demux/2 -> Unit Delay1/1
  Demux/1 -> Terminator/1
  Tx_S/1 -> Demux/1
  Rising edge/1 -> Subsystem1/1
  Logical Operator3/1 -> Subsystem4/1
  AccA_OK/1 -> Logical Operator3/2
  Unit Delay2/1 -> Logical Operator3/1
  Unit Delay1/1 -> Rising edge/1, Unit Delay2/1, Falling edge/1
  Switch/1 -> Divide1/2
  Constant/1 -> Switch/3
  Compare To Zero1/1 -> Logical Operator1/2
  Vector Concatenate2/1 -> Enabled Subsystem1/1(In1)
  Divide1/1 -> Vector Concatenate2/1
  Subsystem1/1 -> Switch/2, Compare To Zero1/1, Switch/1, Vector Concatenate2/3, Sum1/2
  Falling edge/1 -> Logical Operator1/1
  Subsystem4/1 -> Sum1/1
  Sum1/1 -> Vector Concatenate2/2, Divide1/1
  Logical Operator1/1 -> Enabled Subsystem1/Enable
  Enabled Subsystem1/1(Out1) -> Out1/1

== system BLE_Library/Diagnostics/Subsystem2 ==
  In1 : Inport
  In2 : Inport  Port=2
  In3 : Inport  Port=3
  Constant1 : Constant  Value=2402e6  SampleTime=Slot_Ts
  Constant2 : Constant  Value=2412e6  SampleTime=Slot_Ts
  Gain : Gain  Gain=BT_Hop_Separation
  Gain1 : Gain  Gain=BT_Hop_Separation
  Gain2 : Gain  Gain=5e6
  Look-Up Table : Lookup  InputValues=0:39  Table=[1:11 13:38 0 12 39]  SaturateOnIntegerOverflow=on
  Look-Up Table1 : Lookup  InputValues=0:39  Table=[1:11 13:38 0 12 39]  SaturateOnIntegerOverflow=on
  Sum : Sum  Inputs=|++
  Sum1 : Sum  Inputs=|++
  Sum2 : Sum  Inputs=|++
  Out1 : Outport
  Out2 : Outport  Port=2
  Out3 : Outport  Port=3
  wires:
  Sum/1 -> Out1/1
  Look-Up Table/1 -> Gain/1
  Constant1/1 -> Sum1/2, Sum/2
  In1/1 -> Look-Up Table/1
  In2/1 -> Look-Up Table1/1
  Look-Up Table1/1 -> Gain1/1
  Sum1/1 -> Out2/1
  In3/1 -> Gain2/1
  Constant2/1 -> Sum2/2
  Sum2/1 -> Out3/1
  Gain/1 -> Sum/1
  Gain1/1 -> Sum1/1
  Gain2/1 -> Sum2/1

== system BLE_Library/Packet Error Rate/Enabled Subsystem ==
  In1 : Inport
  Enable : EnablePort
  Out1 : Outport
  wires:
  In1/1 -> Out1/1

== system BLE_Library/Packet Rejection Rate/Enabled Subsystem1 ==
  In1 : Inport
  Enable : EnablePort
  Out1 : Outport
  wires:
  In1/1 -> Out1/1

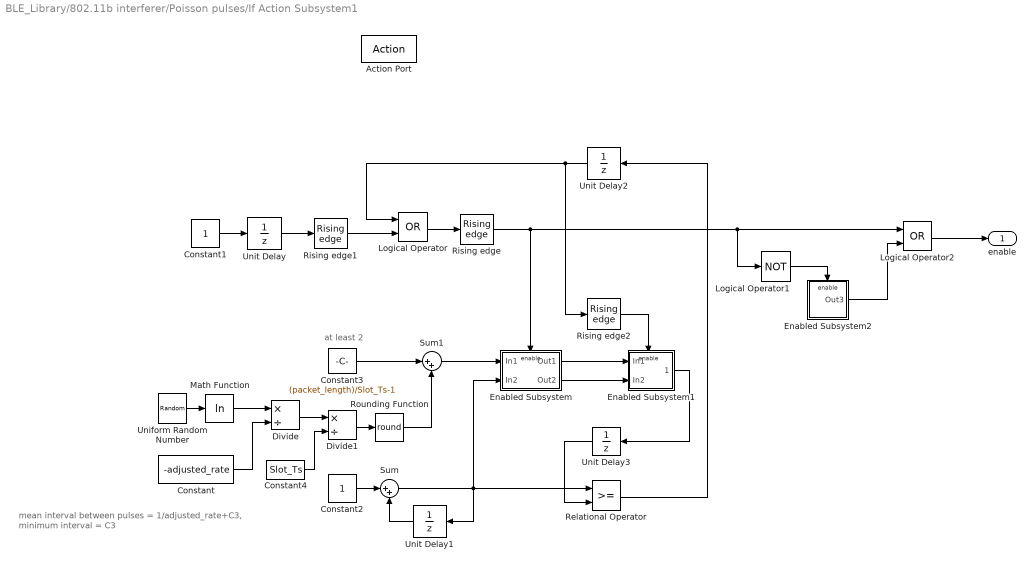
== system BLE_Library/802.11b interferer/Poisson pulses/If Action Subsystem1 ==
  note: at least 2
  note: mean interval between pulses = 1/adjusted_rate+C3,
      | minimum interval = C3
  Action Port : ActionPort  InitializeStates=reset
  Constant : Constant  Value=-adjusted_rate  SampleTime=Slot_Ts
  Constant1 : Constant  SampleTime=Slot_Ts
  Constant2 : Constant  SampleTime=Slot_Ts
  Constant3 : Constant  Value=(packet_length)/Slot_Ts-1  SampleTime=Slot_Ts
  Constant4 : Constant  Value=Slot_Ts  SampleTime=Slot_Ts
  Divide : Product  Inputs=*/
  Divide1 : Product  Inputs=*/
  Enabled Subsystem : Subsystem  TreatAsAtomicUnit=on
  Enabled Subsystem1 : Subsystem  TreatAsAtomicUnit=on
  Enabled Subsystem2 : Subsystem  TreatAsAtomicUnit=on
  Logical Operator : Logic  Operator=OR  AllPortsSameDT=off  OutDataTypeStr=boolean
  Logical Operator1 : Logic  Operator=NOT  AllPortsSameDT=off  OutDataTypeStr=boolean
  Logical Operator2 : Logic  Operator=OR  AllPortsSameDT=off  OutDataTypeStr=boolean
  Math Function : Math  Operator=log  SaturateOnIntegerOverflow=on
  Relational Operator : RelationalOperator  OutDataTypeStr=boolean  RndMeth=Simplest
  Rising edge : BLE_Library/Rising edge  SystemSampleTime=-1
  Rising edge1 : BLE_Library/Rising edge  SystemSampleTime=-1
  Rising edge2 : BLE_Library/Rising edge  SystemSampleTime=-1
  Rounding Function : Rounding  Operator=round
  Sum : Sum  Inputs=|++
  Sum1 : Sum  Inputs=|++
  Uniform Random Number : UniformRandomNumber  Minimum=0  Seed=1  SampleTime=Slot_Ts
  Unit Delay : UnitDelay  SampleTime=Slot_Ts
  Unit Delay1 : UnitDelay  InitialCondition=-1  SampleTime=Slot_Ts
  Unit Delay2 : UnitDelay  SampleTime=Slot_Ts
  Unit Delay3 : UnitDelay  SampleTime=Slot_Ts
  enable : Outport
  wires:
  Logical Operator/1 -> Rising edge/1
  Enabled Subsystem1/1(Out1) -> Unit Delay3/1
  Rising edge1/1 -> Logical Operator/2
  Rising edge2/1 -> Enabled Subsystem1/Enable
  Logical Operator1/1 -> Enabled Subsystem2/Enable
  Unit Delay1/1 -> Sum/2
  Uniform Random Number/1 -> Math Function/1
  Math Function/1 -> Divide/1
  Unit Delay2/1 -> Logical Operator/1, Rising edge2/1
  Constant2/1 -> Sum/1
  Constant1/1 -> Unit Delay/1
  Unit Delay3/1 -> Relational Operator/2
  Enabled Subsystem2/1(Out3) -> Logical Operator2/2
  Divide1/1 -> Rounding Function/1
  Rising edge/1 -> Logical Operator2/1, Logical Operator1/1, Enabled Subsystem/Enable
  Enabled Subsystem/2(Out2) -> Enabled Subsystem1/2(In2)
  Unit Delay/1 -> Rising edge1/1
  Logical Operator2/1 -> enable/1
  Constant3/1 -> Sum1/1
  Divide/1 -> Divide1/1
  Rounding Function/1 -> Sum1/2
  Relational Operator/1 -> Unit Delay2/1
  Sum1/1 -> Enabled Subsystem/1(In1)
  Constant4/1 -> Divide1/2
  Constant/1 -> Divide/2
  Enabled Subsystem/1(Out1) -> Enabled Subsystem1/1(In1)
  Sum/1 -> Unit Delay1/1, Relational Operator/1, Enabled Subsystem/2(In2)

== system BLE_Library/802.11b interferer/Poisson pulses/If Action Subsystem2 ==
  Action Port : ActionPort  InitializeStates=reset
  Constant5 : Constant  OutDataTypeStr=boolean  SampleTime=Slot_Ts
  enable : Outport
  wires:
  Constant5/1 -> enable/1
